simulink model "TEST_FOR_GIT"  (R2024b)
settings: Solver=FixedStepDiscrete  StartTime=0.0  StopTime=10.0  FixedStep=0.001  RelTol=1e-3
settings Model: Creator=415  LastModifiedBy=415
settings OptimizationCC: DefaultParameterBehavior=Inlined  EnhancedBackFolding=on  PassReuseOutputArgsAs=Individual arguments  ZeroExternalMemoryAtStartup=off  ZeroInternalMemoryAtStartup=off  OptimizeBlockOrder=speed  DifferentSizesBufferReuse=on  OptimizationCustomize=off  EfficientTunableParamExpr=on
settings DebuggingCC: ParameterTunabilityLossMsg=error
settings SFSimCC: MATLABDynamicMemAlloc=off
settings RTWCC: Description=Embedded Coder  SystemTargetFile=ert.tlc  TemplateMakefile=ert_default_tmf
settings CodeAppCC: ForceParamTrailComments=on  IgnoreCustomStorageClasses=off  OperatorAnnotations=on  SimulinkDataObjDesc=on  SFDataObjDesc=on  InsertBlockDesc=on
settings ERTTargetCC: TargetLangStandard=C99 (ISO)  GenerateSampleERTMain=on  ERTCustomFileTemplate=example_file_process.tlc

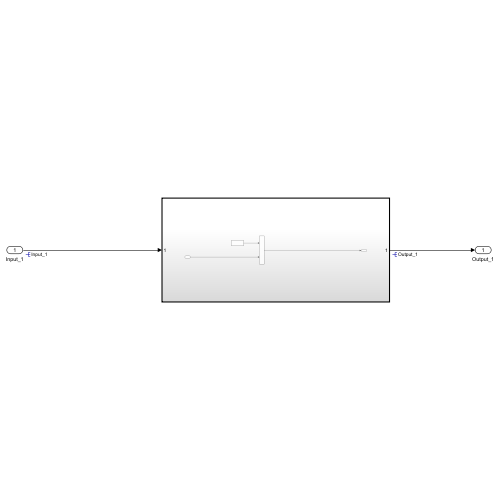
[thumbnail: Simulink's stored preview of the top-level diagram]
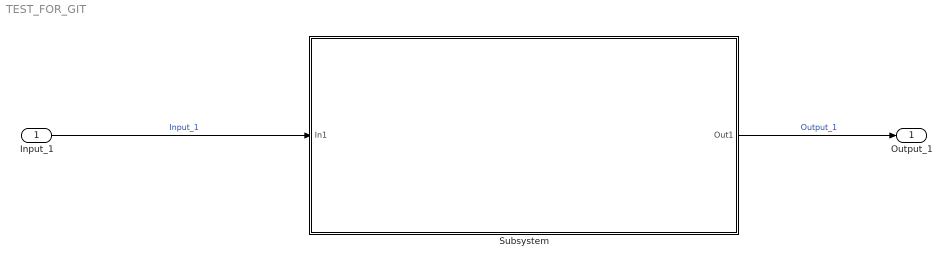
== system TEST_FOR_GIT ==
  Input_1 : Inport
  Subsystem : Subsystem  TreatAsAtomicUnit=on
  Output_1 : Outport
  wires:
  Subsystem/1(Out1) -> Output_1/1  "Output_1"
  Input_1/1 -> Subsystem/1(In1)  "Input_1"

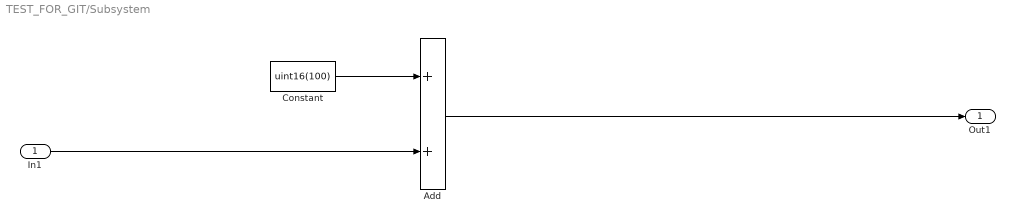
== system TEST_FOR_GIT/Subsystem ==
  In1 : Inport
  Add : Sum
  Constant : Constant  Value=uint16(100)
  Out1 : Outport
  wires:
  Constant/1 -> Add/1
  In1/1 -> Add/2
  Add/1 -> Out1/1
